simulink model "WhippleModel"  (Simulink 7.5)
settings: Solver=ode23s  StartTime=0.0  StopTime=60  RelTol=1e-3
values from neighbouring files (symbols this model uses):
  initialConditions = [0, 0, 0, 0, 0, 0, 0, 0,                       0.0, -speed / par.rR, 0]    [generate_data.m]
  kDelta = gains(1)    [generate_data.m]
  kPhi = gains(3)    [generate_data.m]
  kPhiDot = gains(2)    [generate_data.m]
  kPsi = gains(4)    [generate_data.m]
  kY = gains(5)    [generate_data.m]
  neuroDen = [1, 13.96, 311.85, 2722.5]    [create_ieee_paper_plots.m]    (also in generate_data.m = [1, 2 * .707 * 30, 900])
  neuroNum = 2722.5    [create_ieee_paper_plots.m]    (also in generate_data.m = 900)
  timeDelay = 2.75    [generate_data.m]
undefined symbols (not defined in the file or in its folder): A, B, C, D, gain
libraries: simulink x5
settings Model: Creator=moorepants  LastModifiedBy=moorepants
settings OptimizationCC: InlineParams=on  InlineInvariantSignals=on  InitFltsAndDblsToZero=on
settings DebuggingCC: SaveWithParameterizedLinksMsg=none  SignalResolutionControl=TryResolveAllWithWarning  MultiTaskDSMMsg=warning  MultiTaskCondExecSysMsg=none  StrictBusMsg=None
settings RTWCC: IncludeERTFirstTime=on
settings GRTTargetCC: TargetFcnLib=ansi_tfl_tmw.mat

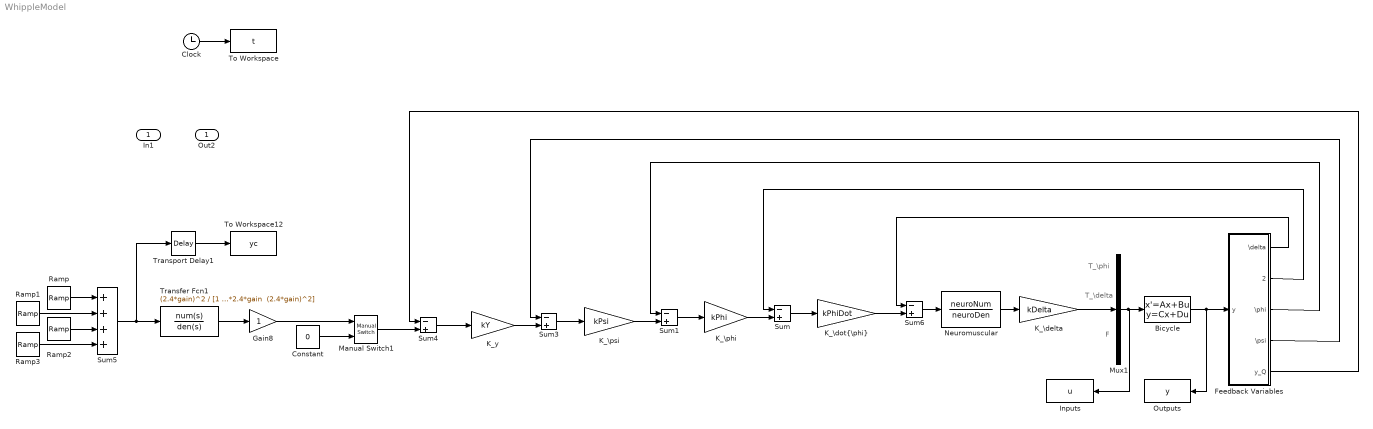
== system WhippleModel ==
  note: T_\phi
  note: T_\delta
  note: F
  In1 : Inport  OutDataType=sfix(16)  OutScaling=2^0
  Bicycle : StateSpace  A=A  B=B  C=C  D=D  X0=initialConditions
  Clock : Clock
      settings: Decimation=10
  Constant : Constant  Value=0  OutDataType=sfix(16)  OutScaling=2^0
  Feedback Variables : Subsystem
  Gain8 : Gain  ParameterDataType=sfix(16)  ParameterScaling=2^0  OutDataType=sfix(16)  OutScaling=2^0
  Inputs : ToWorkspace  VariableName=u  SampleTime=-1  SaveFormat=Array
  K_\delta : Gain  Gain=kDelta  ParameterDataType=sfix(16)  ParameterScaling=2^0  OutDataType=sfix(16)  OutScaling=2^0
  "K_\\dot{\\phi}" : Gain  Gain=kPhiDot  ParameterDataType=sfix(16)  ParameterScaling=2^0  OutDataType=sfix(16)  OutScaling=2^0
  K_\phi : Gain  Gain=kPhi  ParameterDataType=sfix(16)  ParameterScaling=2^0  OutDataType=sfix(16)  OutScaling=2^0
  K_\psi : Gain  Gain=kPsi  ParameterDataType=sfix(16)  ParameterScaling=2^0  OutDataType=sfix(16)  OutScaling=2^0
  K_y : Gain  Gain=kY  ParameterDataType=sfix(16)  ParameterScaling=2^0  OutDataType=sfix(16)  OutScaling=2^0
  Manual Switch1 : simulink/Signal Routing/Manual Switch  SystemSampleTime=-1  sw=1  action=0  varsize=off
  Mux1 : Mux  Inputs=3
  Neuromuscular : TransferFcn  Numerator=neuroNum  Denominator=neuroDen
  Outputs : ToWorkspace  VariableName=y  SampleTime=-1  SaveFormat=Array
  Ramp : simulink/Sources/Ramp  SystemSampleTime=-1  slope=1*7.5/5  start=(7)*5/7.5  X0=0
  Ramp1 : simulink/Sources/Ramp  SystemSampleTime=-1  slope=-1*7.5/5  start=9*5/7.5  X0=0
  Ramp2 : simulink/Sources/Ramp  SystemSampleTime=-1  slope=-1*7.5/5  start=17*5/7.5  X0=0
  Ramp3 : simulink/Sources/Ramp  SystemSampleTime=-1  slope=1*7.5/5  start=19*5/7.5  X0=0
  Sum{,1,3..4,6} (5 alike) : Sum  Inputs=-+  OutDataType=sfix(16)  OutScaling=2^0
  Sum5 : Sum  Inputs=++++  OutDataType=sfix(16)  OutScaling=2^0
  To Workspace : ToWorkspace  VariableName=t  SampleTime=-1  SaveFormat=Array
  To Workspace12 : ToWorkspace  VariableName=yc  SampleTime=-1  SaveFormat=Array
  Transfer Fcn1 : TransferFcn  Numerator=(2.4*gain)^2  Denominator="[1 2*2.4*gain  (2.4*gain)^2]"
  Transport Delay1 : TransportDelay  DelayTime=timeDelay
  Out2 : Outport  OutDataType=sfix(16)  OutScaling=2^0
  wires:
  Sum/1 -> "K_\\dot{\\phi}"/1
  Sum5/1 -> Transfer Fcn1/1, Transport Delay1/1
  Constant/1 -> Manual Switch1/2
  Clock/1 -> To Workspace/1
  Mux1/1 -> Inputs/1, Bicycle/1
  Bicycle/1 -> Outputs/1, Feedback Variables/1(y)
  Ramp/1 -> Sum5/1
  Ramp1/1 -> Sum5/2
  Ramp2/1 -> Sum5/3
  Ramp3/1 -> Sum5/4
  Neuromuscular/1 -> K_\delta/1
  Transfer Fcn1/1 -> Gain8/1
  Sum6/1 -> Neuromuscular/1
  Transport Delay1/1 -> To Workspace12/1
  K_\psi/1 -> Sum1/2
  "K_\\dot{\\phi}"/1 -> Sum6/2
  K_\phi/1 -> Sum/2
  Sum1/1 -> K_\phi/1
  Sum3/1 -> K_\psi/1
  Sum4/1 -> K_y/1
  K_y/1 -> Sum3/2
  Manual Switch1/1 -> Sum4/2
  Gain8/1 -> Manual Switch1/1
  K_\delta/1 -> Mux1/2
  Feedback Variables/1(\delta) -> Sum6/1
  Feedback Variables/2("\\dot{\\phi}") -> Sum/1
  Feedback Variables/3(\phi) -> Sum1/1
  Feedback Variables/4(\psi) -> Sum3/1
  Feedback Variables/5(y_Q) -> Sum4/1

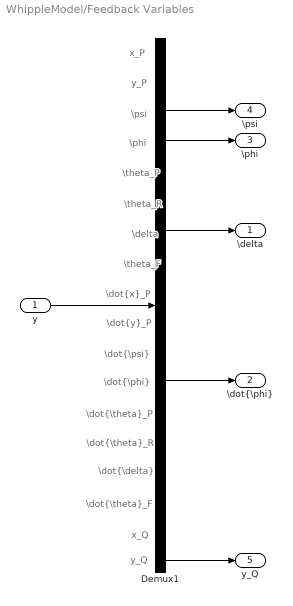
== system WhippleModel/Feedback Variables ==
  note: x_P
  note: y_P
  note: \psi
  note: \phi
  note: \theta_P
  note: \theta_R
  note: \delta
  note: \theta_F
  note: \dot{x}_P
  note: \dot{y}_P
  note: \dot{\psi}
  note: \dot{\phi}
  note: \dot{\theta}_P
  note: \dot{\theta}_R
  note: \dot{\delta}
  note: \dot{\theta}_F
  note: x_Q
  note: y_Q
  y : Inport  OutDataType=fixdt(1, 16)  OutScaling=2^0
  Demux1 : Demux  Outputs=18
  \delta : Outport  OutDataType=fixdt(1, 16)  OutScaling=2^0
  "\\dot{\\phi}" : Outport  Port=2  OutDataType=fixdt(1, 16)  OutScaling=2^0
  \phi : Outport  Port=3  OutDataType=fixdt(1, 16)  OutScaling=2^0
  \psi : Outport  Port=4  OutDataType=fixdt(1, 16)  OutScaling=2^0
  y_Q : Outport  Port=5  OutDataType=fixdt(1, 16)  OutScaling=2^0
  wires:
  y/1 -> Demux1/1
  Demux1/3 -> \psi/1
  Demux1/4 -> \phi/1
  Demux1/7 -> \delta/1
  Demux1/12 -> "\\dot{\\phi}"/1
  Demux1/18 -> y_Q/1
